simulink model "CryoDetHcd"  (R2016b)
settings: Solver=ode45  StartTime=0.0  StopTime=1e-3  RelTol=1e-3
PreLoadFcn:
  | setup_hcd
values from neighbouring files (symbols this model uses):
  A = sqrt(0.5*erfc(x))    [setup_hcd.m]
  Fadc = 307.2e6    (= 307200000)    [setupADCtoDACloopback.m]    (also in setupCryoFPGA_CMB.m; setup_hcd.m = 614000000)
undefined symbols (not defined in the file or in its folder): AXI4, B, C, D, etaRomData, freqRomData, freqRomData1, freqRomData2, freqRomData3, j, Lite
libraries: xbsIndex_r4 x897, CryoDetLibCMB x8, hdlsllib x8, dspsigops x2, simulink x1
(part 1 of 8)
settings Model: Creator=mdewart  LastModifiedBy=mdewart
settings DataIOCC: LimitDataPoints=on  SaveFormat=Array
settings OptimizationCC: BlockReduction=off  BooleanDataType=off  LifeSpan=inf
settings DebuggingCC: SaveWithParameterizedLinksMsg=none  UnderspecifiedInitializationDetection=Classic  MergeDetectMultiDrivingBlocksExec=none  SignalResolutionControl=TryResolveAllWithWarning  SFUnexpectedBacktrackingDiag=warning  SFNoUnconditionalDefaultTransitionDiag=warning  SFExecutionAtInitializationDiag=none
settings HardwareCC: ProdBitPerPointer=32  ProdBitPerSizeT=32  ProdBitPerPtrDiffT=32  ProdLargestAtomicFloat=None  ProdIntDivRoundTo=Undefined  ProdEndianess=Unspecified  ProdWordSize=32  ProdHWDeviceType=32-bit Generic  TargetUnknown=on
settings ModelReferenceCC: PropagateSignalLabelsOutOfModel=off
settings GRTTargetCC: TargetLangStandard=C89/C90 (ANSI)  GeneratePreprocessorConditionals=Disable all
settings ConfigComp: CovMetricSettings=dw  CovHtmlReporting=on  CovSaveCumulativeToWorkspaceVar=on  CovSaveSingleToWorkspaceVar=on  CovExternalEMLEnable=off  CovSFcnEnable=off

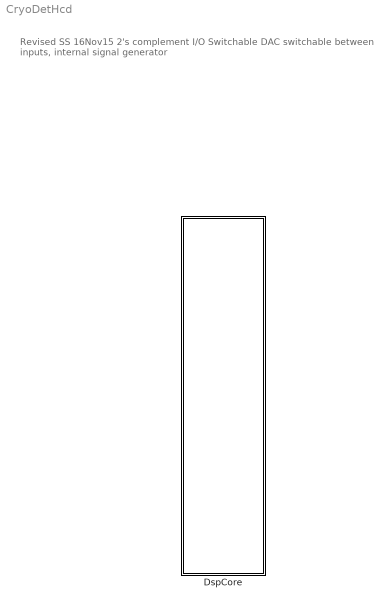
== system CryoDetHcd ==
  note: Revised SS 16Nov15
      | 	2's complement I/O
      | 	Switchable DAC switchable between inputs, internal signal generator
  DspCore : Subsystem

== system CryoDetHcd/DspCore ==
  " System Generator1" : xbsIndex_r4/ System Generator  Tag=genX  xilinxfamily=kintexu  part=xcku060  speed=-2-e  package=ffva1156  synthesis_tool=Vivado  clock_wrapper=Clock Enables  directory=./netlist  proj_type=Vivado  Synth_file=Vivado Synthesis Defaults  Impl_file=Vivado Implementation Defaults  testbench=off  simulink_period=2/Fadc  sysclk_period=2e9/Fadc  dcm_input_clock_period=10  incr_netlist=off  trim_vbits=Everywhere in SubSystem  dbl_ovrd=According to Block Masks  core_generation=According to Block Masks  run_coregen=off  deprecated_control=off  eval_field=0  block_type=sysgen
  DSP : Subsystem
  DSP_axi_lite : Subsystem
  Register{1..13} (13 alike) : xbsIndex_r4/Register  init=0  rst=off  en=off  dbl_ovrd=off  block_type=register
  tag scope: config0=global, config1=global, config2=global, config3=global, config4=global, config6=global, config7=global, config8=global, config=global
  wires:
  DSP_axi_lite/1(config0) -> Register2/1
  Register2/1 -> [config0]
  DSP_axi_lite/2(config1) -> Register1/1
  Register1/1 -> [config1]
  Register3/1 -> [config2]
  DSP_axi_lite/3(config2) -> Register3/1
  Register4/1 -> [config3]
  DSP_axi_lite/4(config3) -> Register4/1
  Register5/1 -> [config4]
  DSP_axi_lite/5(config4) -> Register5/1
  [IQ_status] -> Register6/1
  Register6/1 -> DSP_axi_lite/1(status1)
  [dspCounter] -> Register7/1
  Register7/1 -> DSP_axi_lite/2(status2)
  Register8/1 -> [config]
  DSP_axi_lite/6(config5) -> Register8/1
  [status] -> Register9/1
  Register9/1 -> DSP_axi_lite/3(status3)
  [analysis_IQ] -> Register10/1
  Register10/1 -> DSP_axi_lite/4(status4)
  Register11/1 -> [config6]
  DSP_axi_lite/7(config6) -> Register11/1
  Register12/1 -> [config7]
  DSP_axi_lite/8(config7) -> Register12/1
  DSP_axi_lite/9(config8) -> Register13/1
  Register13/1 -> [config8]

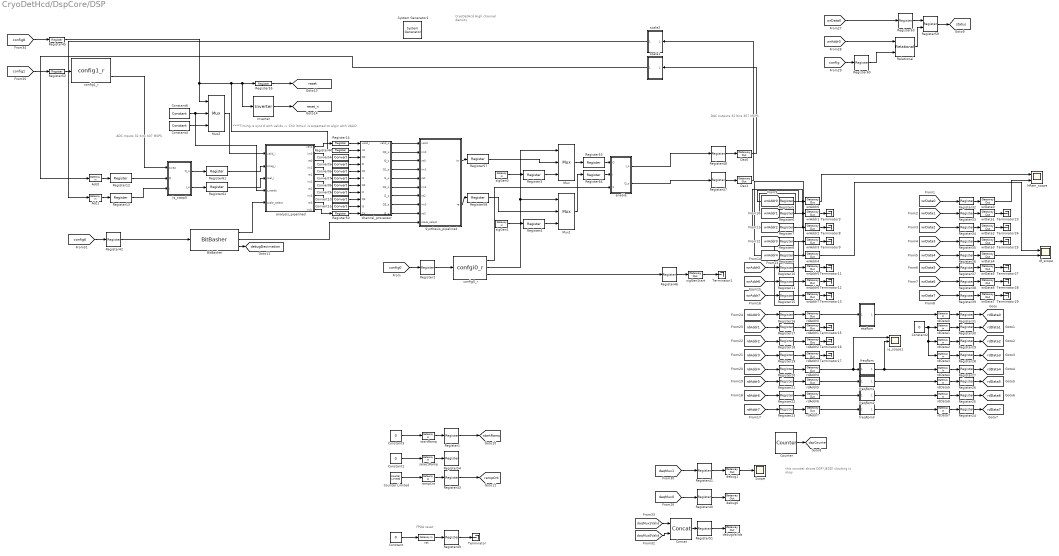
== system CryoDetHcd/DspCore/DSP ==
  note: this counter shows DSP (JESD) clocking
      | is okay
  note: ****Timing is sync'd with valids -> Ch0 (tmux) is expected to algin with VALID
  note: CryoDetHcd
      | High channel density
  note: DAC outputs
      | 32 bits
      | 307 MSPS
  note: ADC Inputs
      | 32 bits
      | 307 MSPS
  note: FPGA reset
  " System Generator1" : xbsIndex_r4/ System Generator  Tag=genX  xilinxfamily=kintexu  part=xcku060  speed=-2-e  package=ffva1156  synthesis_tool=Vivado  clock_wrapper=Clock Enables  directory=./netlist  proj_type=Vivado  Synth_file=Vivado Synthesis Defaults  Impl_file=Vivado Implementation Defaults  testbench=off  simulink_period=2/Fadc  sysclk_period=2e9/Fadc  dcm_input_clock_period=10  incr_netlist=off  trim_vbits=Everywhere in SubSystem  dbl_ovrd=According to Block Masks  core_generation=According to Block Masks  run_coregen=off  deprecated_control=off  eval_field=0  block_type=sysgen
  Adc0 : xbsIndex_r4/Gateway In  gui_display_data_type=Fixed-point  arith_type=Unsigned  n_bits=32  bin_pt=0  preci_type=Single  exp_width=8  frac_width=24  rows=1  columns=1  quantization=Truncate  overflow=Wrap  period=2/Fadc  UseAsADC=off  ADCChannel='1'  interface=None  automatic_assignment=on  address_offset=hex2dec('00')  intf_name=''  intf_description=''  default_value=0  timing_constraint=None  locs_specified=off  LOCs={}  io_standard={}  inherit_from_input=off  hdl_port=on  dbl_ovrd=off  block_type=gatewayin
  Adc1 : xbsIndex_r4/Gateway In  gui_display_data_type=Fixed-point  arith_type=Unsigned  n_bits=32  bin_pt=0  preci_type=Single  exp_width=8  frac_width=24  rows=1  columns=1  quantization=Truncate  overflow=Wrap  period=2/Fadc  UseAsADC=off  ADCChannel='1'  interface=None  automatic_assignment=on  address_offset=hex2dec('00')  intf_name=''  intf_description=''  default_value=0  timing_constraint=None  locs_specified=off  LOCs={}  io_standard={}  inherit_from_input=off  hdl_port=on  dbl_ovrd=off  block_type=gatewayin
  BitBasher : xbsIndex_r4/BitBasher  bitexpr=|  display_expr=off  sr_1=scale_analysis  arith_type1=Unsigned  bin_pt1=0  sr_2=scale_synthesis  arith_type2=Unsigned  bin_pt2=0  sr_3=debugDecimation  arith_type3=Unsigned  bin_pt3=0  sr_4=4  arith_type4=Unsigned  bin_pt4=0  dbl_ovrd=off  block_type=bitbasher
      | scale_analysis = {in[1:0]}
      | scale_synthesis = {in[3:2]}
      | debugDecimation = {in[6:4]}
  Concat : xbsIndex_r4/Concat  num_inputs=2  dbl_ovrd=off  block_type=concat
  Constant{,1..3} (4 alike) : Constant  Value=0
  Constant4 : xbsIndex_r4/Constant  const=0  gui_display_data_type=Boolean  arith_type=Boolean  n_bits=16  bin_pt=14  preci_type=Single  exp_width=8  frac_width=24  explicit_period=on  period=2/Fadc  equ=P=C  opselect=C  inp2=PCIN>>17  opr=+  inp1=P  carry=CIN  dbl_ovrd=off  block_type=constant
  Constant6 : xbsIndex_r4/Constant  const=1.0  gui_display_data_type=Boolean  arith_type=Boolean  n_bits=16  bin_pt=14  preci_type=Single  exp_width=8  frac_width=24  explicit_period=on  period=2/Fadc  equ=P=C  opselect=C  inp2=PCIN>>17  opr=+  inp1=P  carry=CIN  dbl_ovrd=off  block_type=constant
  Convert{4..11} (8 alike) : xbsIndex_r4/Convert  gui_display_data_type=Fixed-point  arith_type="Signed  (2's comp)"  n_bits=16  bin_pt=15  float_type=Single  exp_bits=8  fraction_bits=24  quantization=Truncate  overflow=Saturate  en=off  latency=1  pipeline=off  dbl_ovrd=off  block_type=convert
  Counter : xbsIndex_r4/Counter  cnt_type=Free Running  cnt_to=Inf  operation=Up  start_count=0  cnt_by_val=1  arith_type=Unsigned  n_bits=32  bin_pt=0  load_pin=off  rst=off  en=off  explicit_period=on  period=2/Fadc  use_behavioral_HDL=off  implementation=Fabric  dbl_ovrd=off  block_type=counter
  Counter Limited : simulink/Sources/Counter Limited  uplimit=2^32-1  tsamp=2/Fadc
  Dac0 : xbsIndex_r4/Gateway Out  inherit_from_input=on  hdl_port=on  rows=1  columns=1  UseAsDAC=off  DACChannel='1'  interface=None  automatic_assignment=on  address_offset=hex2dec('00')  intf_name=''  intf_description=''  timing_constraint=None  locs_specified=off  LOCs={}  io_standard={}  block_type=gatewayout
  Dac1 : xbsIndex_r4/Gateway Out  inherit_from_input=on  hdl_port=on  rows=1  columns=1  UseAsDAC=off  DACChannel='1'  interface=None  automatic_assignment=on  address_offset=hex2dec('00')  intf_name=''  intf_description=''  timing_constraint=None  locs_specified=off  LOCs={}  io_standard={}  block_type=gatewayout
  Inverter : xbsIndex_r4/Inverter  en=off  latency=1  dbl_ovrd=off  block_type=inv
  Mux : xbsIndex_r4/Mux  inputs=2  en=off  latency=1  precision=Full  arith_type=Unsigned  n_bits=16  bin_pt=14  quantization=Truncate  overflow=Wrap  dbl_ovrd=off  block_type=mux
  Mux1 : xbsIndex_r4/Mux  inputs=2  en=off  latency=1  precision=Full  arith_type=Unsigned  n_bits=16  bin_pt=14  quantization=Truncate  overflow=Wrap  dbl_ovrd=off  block_type=mux
  Mux2 : xbsIndex_r4/Mux  inputs=2  en=off  latency=1  precision=Full  arith_type=Unsigned  n_bits=16  bin_pt=14  quantization=Truncate  overflow=Wrap  dbl_ovrd=off  block_type=mux
  Register{1..55,57..58,60..64} (62 alike) : xbsIndex_r4/Register  init=0  rst=off  en=off  dbl_ovrd=off  block_type=register
  Register59 : xbsIndex_r4/Register  init=0  rst=off  en=on  dbl_ovrd=off  block_type=register
  Relational : xbsIndex_r4/Relational  mode=a=b  op_type=Bool  en=off  latency=1  dbl_ovrd=off  block_type=relational
  Scope : Scope
  Synthesis_pipelined : Subsystem  VariantControl=Variant
  Terminator{,1,3,8..9,11..13,15..17,23..25,27..29} (17 alike) : Terminator
  analysis_pipelined : Subsystem
  channel_processor : Subsystem  Variant=on  OverrideUsingVariant=Variant
  config0_r : CryoDetLibCMB/confgi0_r
  config1_r : CryoDetLibCMB/config1_r
  debug0 : xbsIndex_r4/Gateway Out  inherit_from_input=on  hdl_port=on  rows=1  columns=1  UseAsDAC=off  DACChannel='1'  interface=None  automatic_assignment=on  address_offset=hex2dec('00')  intf_name=''  intf_description=''  timing_constraint=None  locs_specified=off  LOCs={}  io_standard={}  block_type=gatewayout
  debug1 : xbsIndex_r4/Gateway Out  inherit_from_input=on  hdl_port=on  rows=1  columns=1  UseAsDAC=off  DACChannel='1'  interface=None  automatic_assignment=on  address_offset=hex2dec('00')  intf_name=''  intf_description=''  timing_constraint=None  locs_specified=off  LOCs={}  io_standard={}  block_type=gatewayout
  debugValids : xbsIndex_r4/Gateway Out  inherit_from_input=on  hdl_port=on  rows=1  columns=1  UseAsDAC=off  DACChannel='1'  interface=None  automatic_assignment=on  address_offset=hex2dec('00')  intf_name=''  intf_description=''  timing_constraint=None  locs_specified=off  LOCs={}  io_standard={}  block_type=gatewayout
  df_scope : Scope  NumInputPorts=2
  enable : Subsystem
  etaRom : Subsystem
  freqRom : Subsystem
  freqRom1 : Subsystem
  freqRom2 : Subsystem
  freqRom3 : Subsystem
  iq_scope1 : Scope  NumInputPorts=3
  iq_swap0 : Subsystem
  lrRam_scope : Scope  NumInputPorts=2
  rampCnt : xbsIndex_r4/Gateway In  gui_display_data_type=Fixed-point  arith_type=Unsigned  n_bits=32  bin_pt=0  preci_type=Single  exp_width=8  frac_width=24  rows=1  columns=1  quantization=Truncate  overflow=Wrap  period=2/Fadc  UseAsADC=off  ADCChannel='1'  interface=None  automatic_assignment=on  address_offset=hex2dec('00')  intf_name=''  intf_description=''  default_value=0  timing_constraint=None  locs_specified=off  LOCs={}  io_standard={}  inherit_from_input=off  hdl_port=on  dbl_ovrd=off  block_type=gatewayin
  rdAddr{0..7} (8 alike) : xbsIndex_r4/Gateway Out  inherit_from_input=on  hdl_port=on  rows=1  columns=1  UseAsDAC=off  DACChannel='1'  interface=None  automatic_assignment=on  address_offset=hex2dec('00')  intf_name=''  intf_description=''  timing_constraint=None  locs_specified=off  LOCs={}  io_standard={}  block_type=gatewayout
  rdData{0..7} (8 alike) : xbsIndex_r4/Gateway In  gui_display_data_type=Fixed-point  arith_type=Unsigned  n_bits=32  bin_pt=0  preci_type=Single  exp_width=8  frac_width=24  rows=1  columns=1  quantization=Truncate  overflow=Wrap  period=2/Fadc  UseAsADC=off  ADCChannel='1'  interface=None  automatic_assignment=on  address_offset=hex2dec('00')  intf_name=''  intf_description=''  default_value=0  timing_constraint=None  locs_specified=off  LOCs={}  io_standard={}  inherit_from_input=off  hdl_port=on  dbl_ovrd=off  block_type=gatewayin
  rst : xbsIndex_r4/Gateway In  gui_display_data_type=Boolean  arith_type=Boolean  n_bits=16  bin_pt=14  preci_type=Single  exp_width=8  frac_width=24  rows=1  columns=1  quantization="Round  (unbiased: +/- Inf)"  overflow=Saturate  period=2/Fadc  UseAsADC=off  ADCChannel='1'  interface=None  automatic_assignment=on  address_offset=hex2dec('00')  intf_name=''  intf_description=''  default_value=0  timing_constraint=None  locs_specified=off  LOCs={}  io_standard={}  inherit_from_input=off  hdl_port=on  dbl_ovrd=off  block_type=gatewayin
  scale1 : Subsystem
  scale2 : Subsystem
  selectRamp : xbsIndex_r4/Gateway In  gui_display_data_type=Boolean  arith_type=Boolean  n_bits=16  bin_pt=14  preci_type=Single  exp_width=8  frac_width=24  rows=1  columns=1  quantization=Truncate  overflow=Wrap  period=2/Fadc  UseAsADC=off  ADCChannel='1'  interface=None  automatic_assignment=on  address_offset=hex2dec('00')  intf_name=''  intf_description=''  default_value=0  timing_constraint=None  locs_specified=off  LOCs={}  io_standard={}  inherit_from_input=off  hdl_port=on  dbl_ovrd=off  block_type=gatewayin
  sigGen0 : xbsIndex_r4/Gateway In  gui_display_data_type=Fixed-point  arith_type=Unsigned  n_bits=32  bin_pt=0  preci_type=Single  exp_width=8  frac_width=24  rows=1  columns=1  quantization=Truncate  overflow=Wrap  period=2/Fadc  UseAsADC=off  ADCChannel='1'  interface=None  automatic_assignment=on  address_offset=hex2dec('00')  intf_name=''  intf_description=''  default_value=0  timing_constraint=None  locs_specified=off  LOCs={}  io_standard={}  inherit_from_input=off  hdl_port=on  dbl_ovrd=off  block_type=gatewayin
  sigGen1 : xbsIndex_r4/Gateway In  gui_display_data_type=Fixed-point  arith_type=Unsigned  n_bits=32  bin_pt=0  preci_type=Single  exp_width=8  frac_width=24  rows=1  columns=1  quantization=Truncate  overflow=Wrap  period=2/Fadc  UseAsADC=off  ADCChannel='1'  interface=None  automatic_assignment=on  address_offset=hex2dec('00')  intf_name=''  intf_description=''  default_value=0  timing_constraint=None  locs_specified=off  LOCs={}  io_standard={}  inherit_from_input=off  hdl_port=on  dbl_ovrd=off  block_type=gatewayin
  sigGenStart : xbsIndex_r4/Gateway Out  inherit_from_input=on  hdl_port=on  rows=1  columns=1  UseAsDAC=off  DACChannel='1'  interface=None  automatic_assignment=off  address_offset=hex2dec('004')  intf_name=''  intf_description=''  timing_constraint=None  locs_specified=off  LOCs={}  io_standard={}  block_type=gatewayout
  startRamp : xbsIndex_r4/Gateway In  gui_display_data_type=Boolean  arith_type=Boolean  n_bits=16  bin_pt=14  preci_type=Single  exp_width=8  frac_width=24  rows=1  columns=1  quantization=Truncate  overflow=Wrap  period=2/Fadc  UseAsADC=off  ADCChannel='1'  interface=None  automatic_assignment=on  address_offset=hex2dec('00')  intf_name=''  intf_description=''  default_value=0  timing_constraint=None  locs_specified=off  LOCs={}  io_standard={}  inherit_from_input=off  hdl_port=on  dbl_ovrd=off  block_type=gatewayin
  wrAddr{0..7} (8 alike) : xbsIndex_r4/Gateway Out  inherit_from_input=on  hdl_port=on  rows=1  columns=1  UseAsDAC=off  DACChannel='1'  interface=None  automatic_assignment=on  address_offset=hex2dec('00')  intf_name=''  intf_description=''  timing_constraint=None  locs_specified=off  LOCs={}  io_standard={}  block_type=gatewayout
  wrData{0..7} (8 alike) : xbsIndex_r4/Gateway Out  inherit_from_input=on  hdl_port=on  rows=1  columns=1  UseAsDAC=off  DACChannel='1'  interface=None  automatic_assignment=on  address_offset=hex2dec('00')  intf_name=''  intf_description=''  timing_constraint=None  locs_specified=off  LOCs={}  io_standard={}  block_type=gatewayout
  tag scope: debugDecimation=global, dspCounter=global, rampCnt=global, rdData0=global, rdData1=global, rdData2=global, rdData3=global, rdData4=global, rdData5=global, rdData6=global, rdData7=global, reset=global, reset_n=global, startRamp=global, status=global
  wires:
  startRamp/1 -> Register1/1
  Constant/1 -> rst/1
  rst/1 -> Register49/1
  sigGen0/1 -> Register3/1
  sigGen1/1 -> Register4/1
  sigGenStart/1 -> Terminator1/1
  [config0] -> Register2/1
  Register3/1 -> Mux/3
  Synthesis_pipelined/1(im) -> Register57/1
  Synthesis_pipelined/2(re) -> Register58/1
  analysis_pipelined/1(valid) -> Register14/1
  analysis_pipelined/2(im0) -> Convert4/1
  analysis_pipelined/3(re0) -> Convert5/1
  analysis_pipelined/4(im1) -> Convert6/1
  analysis_pipelined/5(re1) -> Convert7/1
  analysis_pipelined/6(im2) -> Convert8/1
  analysis_pipelined/7(re2) -> Convert9/1
  analysis_pipelined/8(im3) -> Convert10/1
  analysis_pipelined/9(re3) -> Convert11/1
  Adc0/1 -> Register12/1
  Adc1/1 -> Register13/1
  Register4/1 -> Mux1/3
  Register5/1 -> wrAddr0/1
  Register6/1 -> wrAddr1/1
  Register7/1 -> wrAddr2/1
  Register8/1 -> wrAddr3/1
  Register9/1 -> wrAddr4/1
  Register10/1 -> wrAddr5/1
  Register11/1 -> wrAddr6/1
  Register15/1 -> wrAddr7/1
  Register16/1 -> rdAddr0/1
  Register17/1 -> rdAddr1/1
  Register18/1 -> rdAddr2/1
  Register19/1 -> rdAddr3/1
  Register20/1 -> rdAddr4/1
  Register21/1 -> rdAddr5/1
  Register22/1 -> rdAddr6/1
  Register23/1 -> rdAddr7/1
  rdData7/1 -> Register24/1
  rdData3/1 -> Register28/1
  rdData4/1 -> Register27/1
  rdData5/1 -> Register26/1
  rdData6/1 -> Register25/1
  rdData2/1 -> Register29/1
  rdData1/1 -> Register30/1
  rdData0/1 -> Register31/1
  Register32/1 -> wrData0/1
  Register33/1 -> wrData1/1
  Register34/1 -> wrData2/1
  Register35/1 -> wrData3/1
  Register36/1 -> wrData4/1
  Register37/1 -> wrData5/1
  Register38/1 -> wrData6/1
  Register39/1 -> wrData7/1
  Register31/1 -> [rdData0]
  Register30/1 -> [rdData1]
  Register28/1 -> [rdData3]
  Register27/1 -> [rdData4]
  Register25/1 -> [rdData6]
  Register24/1 -> [rdData7]
  Register29/1 -> [rdData2]
  [wrData0] -> Register32/1
  [wrData7] -> Register39/1
  [wrData6] -> Register38/1
  [wrData5] -> Register37/1
  [wrData4] -> Register36/1
  [wrData3] -> Register35/1
  [wrData2] -> Register34/1
  [wrData1] -> Register33/1
  [wrAddr7] -> Register15/1
  [wrAddr6] -> Register11/1
  [wrAddr5] -> Register10/1
  [wrAddr4] -> Register9/1
  [wrAddr3] -> Register8/1
  [wrAddr2] -> Register7/1
  [wrAddr1] -> Register6/1
  [wrAddr0] -> Register5/1
  [rdAddr7] -> Register23/1
  [rdAddr6] -> Register22/1
  [rdAddr5] -> Register21/1
  [rdAddr4] -> Register20/1
  [rdAddr3] -> Register19/1
  [rdAddr2] -> Register18/1
  [rdAddr1] -> Register17/1
  [rdAddr0] -> Register16/1
  wrAddr1/1 -> Terminator3/1
  wrAddr2/1 -> Terminator8/1
  wrAddr3/1 -> Terminator9/1
  wrAddr4/1 -> df_scope/1
  wrAddr5/1 -> Terminator11/1
  wrAddr6/1 -> Terminator12/1
  wrAddr7/1 -> Terminator13/1
  rdAddr1/1 -> Terminator15/1
  rdAddr2/1 -> Terminator16/1
  rdAddr3/1 -> Terminator17/1
  wrData1/1 -> Terminator23/1
  wrData2/1 -> Terminator24/1
  wrData3/1 -> Terminator25/1
  wrData5/1 -> Terminator27/1
  wrData6/1 -> Terminator28/1
  wrData7/1 -> Terminator29/1
  Constant2/1 -> rdData1/1, rdData2/1, rdData3/1
  Register26/1 -> [rdData5]
  Register40/1 -> debug0/1
  Register41/1 -> debug1/1
  Register47/1 -> Dac1/1
  Register48/1 -> Dac0/1
  Register49/1 -> Terminator/1
  Constant3/1 -> startRamp/1
  analysis_pipelined/10(indx) -> Register50/1
  Register51/1 -> debugValids/1
  [config1] -> Register52/1
  Register46/1 -> sigGenStart/1
  Mux/1 -> Register53/1
  config0_r/2 -> Mux1/1, Mux/1
  Register2/1 -> config0_r/1
  config0_r/3 -> Register46/1
  Register52/1 -> config1_r/1
  config1_r/2 -> iq_swap0/1(swap)
  Register12/1 -> iq_swap0/2(Q)
  Register13/1 -> iq_swap0/3(I)
  iq_swap0/1(Q_o) -> Register61/1
  iq_swap0/2(I_o) -> Register62/1
  Counter/1 -> [dspCounter]
  Convert7/1 -> channel_processor/6(I1)
  Convert5/1 -> channel_processor/4(I0)
  Convert10/1 -> channel_processor/9(Q3)
  Convert11/1 -> channel_processor/10(I3)
  Register50/1 -> channel_processor/11(Ch)
  Register14/1 -> channel_processor/1(valid_i)
  Convert9/1 -> channel_processor/8(I2)
  Convert6/1 -> channel_processor/5(Q1)
  Convert4/1 -> channel_processor/3(Q0)
  Convert8/1 -> channel_processor/7(Q2)
  channel_processor/5(I1_o) -> Synthesis_pipelined/5(re1)
  channel_processor/4(Q1_o) -> Synthesis_pipelined/4(im1)
  channel_processor/6(Q2_o) -> Synthesis_pipelined/6(im2)
  channel_processor/7(I2_o) -> Synthesis_pipelined/7(re2)
  channel_processor/8(Q3_o) -> Synthesis_pipelined/8(im3)
  channel_processor/1(valid_o) -> Synthesis_pipelined/1(valid)
  channel_processor/9(I3_o) -> Synthesis_pipelined/9(re3)
  channel_processor/2(Q0_o) -> Synthesis_pipelined/2(im0)
  channel_processor/3(I0_o) -> Synthesis_pipelined/3(re0)
  Register53/1 -> enable/1(Q)
  config0_r/1 -> enable/3(enable)
  Register57/1 -> Mux/2
  Register58/1 -> Mux1/2
  rdAddr4/1 -> iq_scope1/1, freqRom/1(In1)
  freqRom/1(Out1) -> iq_scope1/2, rdData4/1
  wrAddr0/1 -> lrRam_scope/1
  wrData0/1 -> lrRam_scope/2
  wrData4/1 -> df_scope/2
  [wrAddr0] -> Relational/1
  [wrData0] -> Register63/1
  Register59/1 -> [status]
  Register60/1 -> Relational/2
  [config] -> Register60/1
  Register61/1 -> analysis_pipelined/2(imag_i)
  Register62/1 -> analysis_pipelined/3(real_i)
  Relational/1 -> Register59/2
  Register63/1 -> Register59/1
  Dac0/1 -> scale1/1(In1)
  Dac1/1 -> scale2/1(In1)
  scale1/1(Out1) -> Adc0/1
  scale2/1(Out1) -> Adc1/1
  enable/1(I_o) -> Register48/1
  enable/2(Q_o) -> Register47/1
  etaRom/1(Out1) -> rdData0/1
  rdAddr0/1 -> etaRom/1(In1)
  Mux1/1 -> Register64/1
  Register64/1 -> enable/2(I)
  selectRamp/1 -> Register54/1
  Constant1/1 -> selectRamp/1
  Register1/1 -> [startRamp]
  [daqMux0] -> Register40/1
  [daqMux1] -> Register41/1
  [config6] -> Register42/1
  Register42/1 -> BitBasher/1
  BitBasher/2 -> Synthesis_pipelined/10(scale_select)
  BitBasher/1 -> analysis_pipelined/5(scale_select)
  [daqMux1Valid] -> Concat/1
  Concat/1 -> Register51/1
  [daqMux0Valid] -> Concat/2
  BitBasher/3 -> [debugDecimation]
  rampCnt/1 -> Register43/1
  Register43/1 -> [rampCnt]
  rdAddr5/1 -> freqRom1/1(In1)
  freqRom1/1(Out1) -> rdData5/1
  rdAddr6/1 -> freqRom2/1(In1)
  freqRom2/1(Out1) -> rdData6/1
  rdAddr7/1 -> freqRom3/1(In1)
  freqRom3/1(Out1) -> rdData7/1
  debug1/1 -> Scope/1
  Counter Limited/1 -> rampCnt/1
  Register45/1 -> Mux2/1, Register55/1, Inverter/1, Register44/1
  Constant6/1 -> Mux2/2, analysis_pipelined/4(t_ready)
  Mux2/1 -> analysis_pipelined/1(valid_i)
  Constant4/1 -> Mux2/3
  Register44/1 -> channel_processor/2(rst)
  [config8] -> Register45/1
  Inverter/1 -> [reset_n]
  Register55/1 -> [reset]

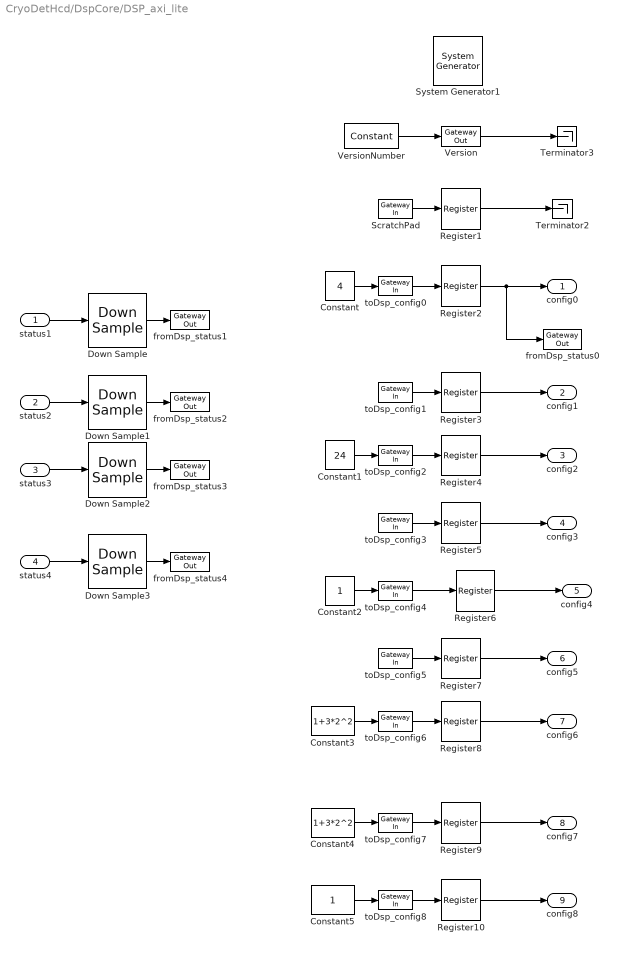
== system CryoDetHcd/DspCore/DSP_axi_lite ==
  status1 : Inport
  status2 : Inport  Port=2
  status3 : Inport  Port=3
  status4 : Inport  Port=4
  " System Generator1" : xbsIndex_r4/ System Generator  Tag=genX  xilinxfamily=kintexu  part=xcku060  speed=-2-e  package=ffva1156  synthesis_tool=Vivado  clock_wrapper=Clock Enables  directory=./netlist  proj_type=Vivado  Synth_file=Vivado Synthesis Defaults  Impl_file=Vivado Implementation Defaults  testbench=off  simulink_period=1/156.25e6  sysclk_period=1e9/(156.25e6)  dcm_input_clock_period=10  incr_netlist=off  trim_vbits=Everywhere in SubSystem  dbl_ovrd=According to Block Masks  core_generation=According to Block Masks  run_coregen=off  deprecated_control=off  eval_field=0  block_type=sysgen
  Constant : Constant  Value=4
  Constant1 : Constant  Value=24
  Constant2 : Constant
  Constant3 : Constant  Value=1+3*2^2
  Constant4 : Constant  Value=1+3*2^2
  Constant5 : Constant
  Down Sample{,1..3} (4 alike) : xbsIndex_r4/Down Sample  sample_ratio=16  sample_phase="Last Value of Frame  (most efficient)"  en=off  rst=off  latency=1  dbl_ovrd=off  block_type=dsamp
  Register{1..10} (10 alike) : xbsIndex_r4/Register  init=0  rst=off  en=off  dbl_ovrd=off  block_type=register
  ScratchPad : xbsIndex_r4/Gateway In  gui_display_data_type=Fixed-point  arith_type=Unsigned  n_bits=32  bin_pt=0  preci_type=Single  exp_width=8  frac_width=24  rows=1  columns=1  quantization="Round  (unbiased: +/- Inf)"  overflow=Saturate  period=16/156.25e6  UseAsADC=off  ADCChannel='1'  interface=AXI4-Lite  automatic_assignment=off  address_offset=hex2dec('FFC')  intf_name=''  intf_description=''  default_value=0  timing_constraint=None  locs_specified=off  LOCs={}  io_standard={}  inherit_from_input=off  hdl_port=on  dbl_ovrd=off  block_type=gatewayin
  Terminator2 : Terminator
  Terminator3 : Terminator
  Version : xbsIndex_r4/Gateway Out  inherit_from_input=on  hdl_port=on  rows=1  columns=1  UseAsDAC=off  DACChannel='1'  interface=AXI4-Lite  automatic_assignment=off  address_offset=hex2dec('000')  intf_name=''  intf_description=''  timing_constraint=None  locs_specified=off  LOCs={}  io_standard={}  block_type=gatewayout
  VersionNumber : xbsIndex_r4/Constant  const=hex2dec('00000001')  gui_display_data_type=Fixed-point  arith_type=Unsigned  n_bits=32  bin_pt=0  preci_type=Single  exp_width=8  frac_width=24  explicit_period=on  period=16/156.25e6  equ=P=C  opselect=C  inp2=PCIN>>17  opr=+  inp1=P  carry=CIN  dbl_ovrd=off  block_type=constant
  fromDsp_status0 : xbsIndex_r4/Gateway Out  inherit_from_input=on  hdl_port=on  rows=1  columns=1  UseAsDAC=off  DACChannel='1'  interface=AXI4-Lite  automatic_assignment=off  address_offset=hex2dec('004')  intf_name=''  intf_description=''  timing_constraint=None  locs_specified=off  LOCs={}  io_standard={}  block_type=gatewayout
  fromDsp_status1 : xbsIndex_r4/Gateway Out  inherit_from_input=on  hdl_port=on  rows=1  columns=1  UseAsDAC=off  DACChannel='1'  interface=AXI4-Lite  automatic_assignment=off  address_offset=hex2dec('008')  intf_name=''  intf_description=''  timing_constraint=None  locs_specified=off  LOCs={}  io_standard={}  block_type=gatewayout
  fromDsp_status2 : xbsIndex_r4/Gateway Out  inherit_from_input=on  hdl_port=on  rows=1  columns=1  UseAsDAC=off  DACChannel='1'  interface=AXI4-Lite  automatic_assignment=off  address_offset=hex2dec('00C')  intf_name=''  intf_description=''  timing_constraint=None  locs_specified=off  LOCs={}  io_standard={}  block_type=gatewayout
  fromDsp_status3 : xbsIndex_r4/Gateway Out  inherit_from_input=on  hdl_port=on  rows=1  columns=1  UseAsDAC=off  DACChannel='1'  interface=AXI4-Lite  automatic_assignment=off  address_offset=hex2dec('010')  intf_name=''  intf_description=''  timing_constraint=None  locs_specified=off  LOCs={}  io_standard={}  block_type=gatewayout
  fromDsp_status4 : xbsIndex_r4/Gateway Out  inherit_from_input=on  hdl_port=on  rows=1  columns=1  UseAsDAC=off  DACChannel='1'  interface=AXI4-Lite  automatic_assignment=off  address_offset=hex2dec('014')  intf_name=''  intf_description=''  timing_constraint=None  locs_specified=off  LOCs={}  io_standard={}  block_type=gatewayout
  toDsp_config0 : xbsIndex_r4/Gateway In  gui_display_data_type=Fixed-point  arith_type=Unsigned  n_bits=32  bin_pt=0  preci_type=Single  exp_width=8  frac_width=24  rows=1  columns=1  quantization="Round  (unbiased: +/- Inf)"  overflow=Saturate  period=16/156.25e6  UseAsADC=off  ADCChannel='1'  interface=AXI4-Lite  automatic_assignment=off  address_offset=hex2dec('080')  intf_name=''  intf_description=''  default_value=0  timing_constraint=None  locs_specified=off  LOCs={}  io_standard={}  inherit_from_input=off  hdl_port=on  dbl_ovrd=off  block_type=gatewayin
  toDsp_config1 : xbsIndex_r4/Gateway In  gui_display_data_type=Fixed-point  arith_type=Unsigned  n_bits=32  bin_pt=0  preci_type=Single  exp_width=8  frac_width=24  rows=1  columns=1  quantization="Round  (unbiased: +/- Inf)"  overflow=Saturate  period=16/156.25e6  UseAsADC=off  ADCChannel='1'  interface=AXI4-Lite  automatic_assignment=off  address_offset=hex2dec('084')  intf_name=''  intf_description=''  default_value=0  timing_constraint=None  locs_specified=off  LOCs={}  io_standard={}  inherit_from_input=off  hdl_port=on  dbl_ovrd=off  block_type=gatewayin
  toDsp_config2 : xbsIndex_r4/Gateway In  gui_display_data_type=Fixed-point  arith_type=Unsigned  n_bits=32  bin_pt=0  preci_type=Single  exp_width=8  frac_width=24  rows=1  columns=1  quantization="Round  (unbiased: +/- Inf)"  overflow=Saturate  period=16/156.25e6  UseAsADC=off  ADCChannel='1'  interface=AXI4-Lite  automatic_assignment=off  address_offset=hex2dec('088')  intf_name=''  intf_description=''  default_value=0  timing_constraint=None  locs_specified=off  LOCs={}  io_standard={}  inherit_from_input=off  hdl_port=on  dbl_ovrd=off  block_type=gatewayin
  toDsp_config3 : xbsIndex_r4/Gateway In  gui_display_data_type=Fixed-point  arith_type=Unsigned  n_bits=32  bin_pt=0  preci_type=Single  exp_width=8  frac_width=24  rows=1  columns=1  quantization="Round  (unbiased: +/- Inf)"  overflow=Saturate  period=16/156.25e6  UseAsADC=off  ADCChannel='1'  interface=AXI4-Lite  automatic_assignment=off  address_offset=hex2dec('08C')  intf_name=''  intf_description=''  default_value=0  timing_constraint=None  locs_specified=off  LOCs={}  io_standard={}  inherit_from_input=off  hdl_port=on  dbl_ovrd=off  block_type=gatewayin
  toDsp_config4 : xbsIndex_r4/Gateway In  gui_display_data_type=Fixed-point  arith_type=Unsigned  n_bits=16  bin_pt=15  preci_type=Single  exp_width=8  frac_width=24  rows=1  columns=1  quantization="Round  (unbiased: +/- Inf)"  overflow=Saturate  period=16/156.25e6  UseAsADC=off  ADCChannel='1'  interface=AXI4-Lite  automatic_assignment=off  address_offset=hex2dec('090')  intf_name=''  intf_description=''  default_value=0  timing_constraint=None  locs_specified=off  LOCs={}  io_standard={}  inherit_from_input=off  hdl_port=on  dbl_ovrd=off  block_type=gatewayin
  toDsp_config5 : xbsIndex_r4/Gateway In  gui_display_data_type=Fixed-point  arith_type=Unsigned  n_bits=7  bin_pt=0  preci_type=Single  exp_width=8  frac_width=24  rows=1  columns=1  quantization="Round  (unbiased: +/- Inf)"  overflow=Saturate  period=16/156.25e6  UseAsADC=off  ADCChannel='1'  interface=AXI4-Lite  automatic_assignment=off  address_offset=hex2dec('094')  intf_name=''  intf_description=''  default_value=0  timing_constraint=None  locs_specified=off  LOCs={}  io_standard={}  inherit_from_input=off  hdl_port=on  dbl_ovrd=off  block_type=gatewayin
  toDsp_config6 : xbsIndex_r4/Gateway In  gui_display_data_type=Fixed-point  arith_type=Unsigned  n_bits=32  bin_pt=0  preci_type=Single  exp_width=8  frac_width=24  rows=1  columns=1  quantization="Round  (unbiased: +/- Inf)"  overflow=Saturate  period=16/156.25e6  UseAsADC=off  ADCChannel='1'  interface=AXI4-Lite  automatic_assignment=off  address_offset=hex2dec('098')  intf_name=''  intf_description=''  default_value=0  timing_constraint=None  locs_specified=off  LOCs={}  io_standard={}  inherit_from_input=off  hdl_port=on  dbl_ovrd=off  block_type=gatewayin
  toDsp_config7 : xbsIndex_r4/Gateway In  gui_display_data_type=Fixed-point  arith_type=Unsigned  n_bits=32  bin_pt=0  preci_type=Single  exp_width=8  frac_width=24  rows=1  columns=1  quantization="Round  (unbiased: +/- Inf)"  overflow=Saturate  period=16/156.25e6  UseAsADC=off  ADCChannel='1'  interface=AXI4-Lite  automatic_assignment=off  address_offset=hex2dec('09C')  intf_name=''  intf_description=''  default_value=0  timing_constraint=None  locs_specified=off  LOCs={}  io_standard={}  inherit_from_input=off  hdl_port=on  dbl_ovrd=off  block_type=gatewayin
  toDsp_config8 : xbsIndex_r4/Gateway In  gui_display_data_type=Boolean  arith_type=Boolean  n_bits=1  bin_pt=0  preci_type=Single  exp_width=8  frac_width=24  rows=1  columns=1  quantization="Round  (unbiased: +/- Inf)"  overflow=Saturate  period=16/156.25e6  UseAsADC=off  ADCChannel='1'  interface=AXI4-Lite  automatic_assignment=off  address_offset=hex2dec('100')  intf_name=''  intf_description=''  default_value=1  timing_constraint=None  locs_specified=off  LOCs={}  io_standard={}  inherit_from_input=off  hdl_port=on  dbl_ovrd=off  block_type=gatewayin
  config0 : Outport
  config1 : Outport  Port=2
  config2 : Outport  Port=3
  config3 : Outport  Port=4
  config4 : Outport  Port=5
  config5 : Outport  Port=6
  config6 : Outport  Port=7
  config7 : Outport  Port=8
  config8 : Outport  Port=9
  wires:
  toDsp_config0/1 -> Register2/1
  Register2/1 -> config0/1, fromDsp_status0/1
  ScratchPad/1 -> Register1/1
  Version/1 -> Terminator3/1
  VersionNumber/1 -> Version/1
  Register1/1 -> Terminator2/1
  toDsp_config1/1 -> Register3/1
  Register3/1 -> config1/1
  toDsp_config2/1 -> Register4/1
  Register4/1 -> config2/1
  toDsp_config3/1 -> Register5/1
  Register5/1 -> config3/1
  toDsp_config4/1 -> Register6/1
  Register6/1 -> config4/1
  status1/1 -> Down Sample/1
  Down Sample/1 -> fromDsp_status1/1
  status2/1 -> Down Sample1/1
  Down Sample1/1 -> fromDsp_status2/1
  status3/1 -> Down Sample2/1
  Down Sample2/1 -> fromDsp_status3/1
  toDsp_config5/1 -> Register7/1
  Register7/1 -> config5/1
  Constant/1 -> toDsp_config0/1
  Constant1/1 -> toDsp_config2/1
  status4/1 -> Down Sample3/1
  Down Sample3/1 -> fromDsp_status4/1
  Constant2/1 -> toDsp_config4/1
  toDsp_config6/1 -> Register8/1
  Register8/1 -> config6/1
  Constant3/1 -> toDsp_config6/1
  toDsp_config7/1 -> Register9/1
  Register9/1 -> config7/1
  Constant4/1 -> toDsp_config7/1
  toDsp_config8/1 -> Register10/1
  Register10/1 -> config8/1
  Constant5/1 -> toDsp_config8/1

== system CryoDetHcd/DspCore/DSP/Synthesis_pipelined ==
  note: TODO check scale values at bitbashers in synth
  valid : Inport
  im0 : Inport  Port=2
  re0 : Inport  Port=3
  im1 : Inport  Port=4
  re1 : Inport  Port=5
  im2 : Inport  Port=6
  re2 : Inport  Port=7
  im3 : Inport  Port=8
  re3 : Inport  Port=9
  scale_select : Inport  Port=10
  Synthesis : Subsystem
  im : Outport
  re : Outport  Port=2
  wires:
  valid/1 -> Synthesis/1(valid)
  im0/1 -> Synthesis/2(im0)
  im1/1 -> Synthesis/4(im1)
  re2/1 -> Synthesis/7(re2)
  re3/1 -> Synthesis/9(re3)
  re0/1 -> Synthesis/3(re0)
  re1/1 -> Synthesis/5(re1)
  im2/1 -> Synthesis/6(im2)
  im3/1 -> Synthesis/8(im3)
  Synthesis/2(re) -> re/1
  Synthesis/1(im) -> im/1
  scale_select/1 -> Synthesis/10(scale_select)

== system CryoDetHcd/DspCore/DSP/analysis_pipelined ==
  valid_i : Inport
  imag_i : Inport  Port=2
  real_i : Inport  Port=3
  t_ready : Inport  Port=4
  scale_select : Inport  Port=5
  Analysis0 : Subsystem
  Analysis1 : Subsystem
  Demux : Demux  Outputs=8
  Enabled Subsystem : Subsystem  TreatAsAtomicUnit=on
  Gateway Out : xbsIndex_r4/Gateway Out  inherit_from_input=off  hdl_port=off  rows=1  columns=1  UseAsDAC=off  DACChannel='1'  interface=None  automatic_assignment=on  address_offset=hex2dec('00')  intf_name=''  intf_description=''  timing_constraint=None  locs_specified=off  LOCs={}  io_standard={}  block_type=gatewayout
  Gateway Out1 : xbsIndex_r4/Gateway Out  inherit_from_input=off  hdl_port=off  rows=1  columns=1  UseAsDAC=off  DACChannel='1'  interface=None  automatic_assignment=on  address_offset=hex2dec('00')  intf_name=''  intf_description=''  timing_constraint=None  locs_specified=off  LOCs={}  io_standard={}  block_type=gatewayout
  Pre-Analysis0 : Subsystem
  Pre-Analysis1 : Subsystem
  Real-Imag to Complex2 : RealImagToComplex
  Scope : Scope  NumInputPorts=8
  valid : Outport
  im0 : Outport  Port=2
  re0 : Outport  Port=3
  im1 : Outport  Port=4
  re1 : Outport  Port=5
  im2 : Outport  Port=6
  re2 : Outport  Port=7
  im3 : Outport  Port=8
  re3 : Outport  Port=9
  indx : Outport  Port=10
  wires:
  Analysis0/5(valid1) -> Enabled Subsystem/Enable
  Analysis0/6(re1) -> im1/1
  Analysis0/7(im1) -> re1/1
  Demux/1 -> Scope/1
  Demux/2 -> Scope/2
  Demux/3 -> Scope/3
  Demux/4 -> Scope/4
  Demux/5 -> Scope/5
  Demux/6 -> Scope/6
  Demux/7 -> Scope/7
  Demux/8 -> Scope/8
  Enabled Subsystem/1(Out1) -> Demux/1
  Gateway Out1/1 -> Real-Imag to Complex2/1
  Gateway Out/1 -> Real-Imag to Complex2/2
  Real-Imag to Complex2/1 -> Enabled Subsystem/1(In1)
  Analysis1/7(im1) -> re3/1, Gateway Out/1
  Analysis1/6(re1) -> im3/1, Gateway Out1/1
  Analysis1/3(im0) -> re2/1
  Analysis1/2(re0) -> im2/1
  Analysis0/1(valid0) -> valid/1
  Analysis0/2(re0) -> im0/1
  Analysis0/3(im0) -> re0/1
  Pre-Analysis0/3(reo) -> Analysis0/3(In3)
  Pre-Analysis0/2(im0) -> Analysis0/2(In2)
  Pre-Analysis0/1(valid0) -> Analysis0/1(In1)
  t_ready/1 -> Analysis1/4(t_ready), Analysis0/4(t_ready)
  Pre-Analysis1/1(valid0) -> Analysis1/1(In1)
  valid_i/1 -> Pre-Analysis0/1(valid), Pre-Analysis1/1(valid)
  real_i/1 -> Pre-Analysis1/3(re), Pre-Analysis0/3(re)
  imag_i/1 -> Pre-Analysis1/2(im), Pre-Analysis0/2(im)
  Analysis0/4(indx0) -> indx/1
  Pre-Analysis1/2(im0) -> Analysis1/2(In2)
  Pre-Analysis1/3(reo) -> Analysis1/3(In3)
  scale_select/1 -> Analysis1/5(sel_scale), Analysis0/5(sel_scale)

== system CryoDetHcd/DspCore/DSP/channel_processor ==
  note: 1) Add Subsystem or Model blocks as valid variant choices.
      | 2) You cannot connect blocks at this level. At simulation, connectivity is automatically
      | determined, based on the active variant and port name matching.
  valid_i : Inport
  rst : Inport  Port=2
  Q0 : Inport  Port=3
  I0 : Inport  Port=4
  Q1 : Inport  Port=5
  I1 : Inport  Port=6
  Q2 : Inport  Port=7
  I2 : Inport  Port=8
  Q3 : Inport  Port=9
  I3 : Inport  Port=10
  Ch : Inport  Port=11
  channel_processor_x1 : Subsystem  VariantControl=Variant1
  channel_processor_x4 : Subsystem  VariantControl=Variant
  valid_o : Outport
  Q0_o : Outport  Port=2
  I0_o : Outport  Port=3
  Q1_o : Outport  Port=4
  I1_o : Outport  Port=5
  Q2_o : Outport  Port=6
  I2_o : Outport  Port=7
  Q3_o : Outport  Port=8
  I3_o : Outport  Port=9

== system CryoDetHcd/DspCore/DSP/enable ==
  Q : Inport
  I : Inport  Port=2
  enable : Inport  Port=3
  Constant7 : xbsIndex_r4/Constant  const=0  gui_display_data_type=Fixed-point  arith_type=Unsigned  n_bits=32  bin_pt=0  preci_type=Single  exp_width=8  frac_width=24  explicit_period=off  period=1  equ=P=C  opselect=C  inp2=PCIN>>17  opr=+  inp1=P  carry=CIN  dbl_ovrd=off  block_type=constant
  Mux2 : xbsIndex_r4/Mux  inputs=2  en=off  latency=1  precision=Full  arith_type=Unsigned  n_bits=16  bin_pt=14  quantization=Truncate  overflow=Wrap  dbl_ovrd=off  block_type=mux
  Mux3 : xbsIndex_r4/Mux  inputs=2  en=off  latency=1  precision=Full  arith_type=Unsigned  n_bits=16  bin_pt=14  quantization=Truncate  overflow=Wrap  dbl_ovrd=off  block_type=mux
  I_o : Outport
  Q_o : Outport  Port=2
  wires:
  Mux3/1 -> Q_o/1
  Mux2/1 -> I_o/1
  I/1 -> Mux3/3
  Q/1 -> Mux2/3
  enable/1 -> Mux3/1, Mux2/1
  Constant7/1 -> Mux3/2, Mux2/2

== system CryoDetHcd/DspCore/DSP/etaRom ==
  In1 : Inport
  1-D Lookup Table : Lookup_n-D  NumberOfTableDimensions=1  BreakpointsSpecification=Even spacing  BreakpointsForDimension1=[-5:5]  Table=etaRomData  InterpMethod=Nearest  InternalRulePriority=Speed  OutDataTypeStr=uint32  RndMeth=Simplest  InputSameDT=on
  Add : Sum
  Constant16 : Constant
  Delay9 : Delay  InitialCondition=0
  Out1 : Outport
  wires:
  Delay9/1 -> Add/1
  Constant16/1 -> Add/2
  Add/1 -> 1-D Lookup Table/1
  1-D Lookup Table/1 -> Out1/1
  In1/1 -> Delay9/1

== system CryoDetHcd/DspCore/DSP/freqRom ==
  In1 : Inport
  1-D Lookup Table : Lookup_n-D  NumberOfTableDimensions=1  BreakpointsSpecification=Even spacing  BreakpointsForDimension1=[-5:5]  Table=freqRomData  InterpMethod=Nearest  InternalRulePriority=Speed  OutDataTypeStr=uint32  RndMeth=Simplest  InputSameDT=on
  Add : Sum
  Constant16 : Constant
  Delay9 : Delay  InitialCondition=0
  Out1 : Outport
  wires:
  In1/1 -> Delay9/1
  1-D Lookup Table/1 -> Out1/1
  Add/1 -> 1-D Lookup Table/1
  Constant16/1 -> Add/2
  Delay9/1 -> Add/1

== system CryoDetHcd/DspCore/DSP/freqRom1 ==
  In1 : Inport
  1-D Lookup Table : Lookup_n-D  NumberOfTableDimensions=1  BreakpointsSpecification=Even spacing  BreakpointsForDimension1=[-5:5]  Table=freqRomData1  InterpMethod=Nearest  InternalRulePriority=Speed  OutDataTypeStr=uint32  RndMeth=Simplest  InputSameDT=on
  Add : Sum
  Constant16 : Constant
  Delay9 : Delay  InitialCondition=0
  Out1 : Outport
  wires:
  Delay9/1 -> Add/1
  Constant16/1 -> Add/2
  Add/1 -> 1-D Lookup Table/1
  1-D Lookup Table/1 -> Out1/1
  In1/1 -> Delay9/1

== system CryoDetHcd/DspCore/DSP/freqRom2 ==
  In1 : Inport
  1-D Lookup Table : Lookup_n-D  NumberOfTableDimensions=1  BreakpointsSpecification=Even spacing  BreakpointsForDimension1=[-5:5]  Table=freqRomData2  InterpMethod=Nearest  InternalRulePriority=Speed  OutDataTypeStr=uint32  RndMeth=Simplest  InputSameDT=on
  Add : Sum
  Constant16 : Constant
  Delay9 : Delay  InitialCondition=0
  Out1 : Outport
  wires:
  In1/1 -> Delay9/1
  1-D Lookup Table/1 -> Out1/1
  Add/1 -> 1-D Lookup Table/1
  Constant16/1 -> Add/2
  Delay9/1 -> Add/1

== system CryoDetHcd/DspCore/DSP/freqRom3 ==
  In1 : Inport
  1-D Lookup Table : Lookup_n-D  NumberOfTableDimensions=1  BreakpointsSpecification=Even spacing  BreakpointsForDimension1=[-5:5]  Table=freqRomData3  InterpMethod=Nearest  InternalRulePriority=Speed  OutDataTypeStr=uint32  RndMeth=Simplest  InputSameDT=on
  Add : Sum
  Constant16 : Constant
  Delay9 : Delay  InitialCondition=0
  Out1 : Outport
  wires:
  Delay9/1 -> Add/1
  Constant16/1 -> Add/2
  Add/1 -> 1-D Lookup Table/1
  1-D Lookup Table/1 -> Out1/1
  In1/1 -> Delay9/1

== system CryoDetHcd/DspCore/DSP/iq_swap0 ==
  swap : Inport
  Q : Inport  Port=2
  I : Inport  Port=3
  Mux4 : xbsIndex_r4/Mux  inputs=2  en=off  latency=1  precision=Full  arith_type=Unsigned  n_bits=16  bin_pt=14  quantization=Truncate  overflow=Wrap  dbl_ovrd=off  block_type=mux
  Mux5 : xbsIndex_r4/Mux  inputs=2  en=off  latency=1  precision=Full  arith_type=Unsigned  n_bits=16  bin_pt=14  quantization=Truncate  overflow=Wrap  dbl_ovrd=off  block_type=mux
  Q_o : Outport
  I_o : Outport  Port=2
  wires:
  Mux4/1 -> Q_o/1
  Mux5/1 -> I_o/1
  Q/1 -> Mux4/2, Mux5/3
  swap/1 -> Mux5/1, Mux4/1
  I/1 -> Mux5/2, Mux4/3

== system CryoDetHcd/DspCore/DSP/scale1 ==
  In1 : Inport
  Bit Concat : hdlsllib/HDL Operations/Bit Concat  numInputs=2
  Bit Slice : hdlsllib/HDL Operations/Bit Slice  lidx=15  ridx=0
  Bit Slice1 : hdlsllib/HDL Operations/Bit Slice  lidx=31  ridx=16
  Data Type Conversion : DataTypeConversion  OutDataTypeStr=int16  ConvertRealWorld=Stored Integer (SI)
  Data Type Conversion1 : DataTypeConversion  OutDataTypeStr=int16  ConvertRealWorld=Stored Integer (SI)
  Gain : Gain  Gain=1/10  OutDataTypeStr=int16
  Gain1 : Gain  Gain=1/10  OutDataTypeStr=int16
  iq_scale_scope : Scope  NumInputPorts=2
  Out1 : Outport
  wires:
  Gain1/1 -> Bit Concat/2, iq_scale_scope/1
  In1/1 -> Bit Slice1/1, Bit Slice/1
  Bit Slice/1 -> Data Type Conversion/1
  Data Type Conversion/1 -> Gain/1
  Data Type Conversion1/1 -> Gain1/1
  Bit Concat/1 -> Out1/1
  Gain/1 -> Bit Concat/1, iq_scale_scope/2
  Bit Slice1/1 -> Data Type Conversion1/1

== system CryoDetHcd/DspCore/DSP/scale2 ==
  In1 : Inport
  Bit Concat : hdlsllib/HDL Operations/Bit Concat  numInputs=2
  Bit Slice : hdlsllib/HDL Operations/Bit Slice  lidx=15  ridx=0
  Bit Slice1 : hdlsllib/HDL Operations/Bit Slice  lidx=31  ridx=16
  Data Type Conversion : DataTypeConversion  OutDataTypeStr=int16  ConvertRealWorld=Stored Integer (SI)
  Data Type Conversion1 : DataTypeConversion  OutDataTypeStr=int16  ConvertRealWorld=Stored Integer (SI)
  Gain : Gain  Gain=1/10  OutDataTypeStr=int16
  Gain1 : Gain  Gain=1/10  OutDataTypeStr=int16
  iq_scale_scope : Scope  NumInputPorts=2
  Out1 : Outport
  wires:
  Bit Slice1/1 -> Data Type Conversion1/1
  Gain/1 -> iq_scale_scope/2, Bit Concat/1
  Bit Concat/1 -> Out1/1
  Data Type Conversion1/1 -> Gain1/1
  Data Type Conversion/1 -> Gain/1
  Bit Slice/1 -> Data Type Conversion/1
  In1/1 -> Bit Slice/1, Bit Slice1/1
  Gain1/1 -> iq_scale_scope/1, Bit Concat/2

== system CryoDetHcd/DspCore/DSP/Synthesis_pipelined/Synthesis ==
  valid : Inport
  im0 : Inport  Port=2
  re0 : Inport  Port=3
  im1 : Inport  Port=4
  re1 : Inport  Port=5
  im2 : Inport  Port=6
  re2 : Inport  Port=7
  im3 : Inport  Port=8
  re3 : Inport  Port=9
  scale_select : Inport  Port=10
  Combine : Subsystem
  Post_synthesis0 : Subsystem
  Post_sytnehsis1 : Subsystem
  Syntehsis0 : Subsystem
  Syntehsis1 : Subsystem
  im : Outport
  re : Outport  Port=2
  wires:
  Syntehsis0/1(valid_o) -> Post_synthesis0/1(valid)
  Combine/3(re_o) -> re/1
  Post_sytnehsis1/3(reo) -> Combine/5(re1)
  Post_sytnehsis1/2(im0) -> Combine/4(im1)
  Post_synthesis0/3(reo) -> Combine/3(re0)
  Post_synthesis0/2(im0) -> Combine/2(im0)
  Post_synthesis0/1(valid0) -> Combine/1(valid)
  Syntehsis0/3(re0) -> Post_synthesis0/3(re)
  Syntehsis0/2(im0) -> Post_synthesis0/2(im)
  Syntehsis1/1(valid_o) -> Post_sytnehsis1/1(valid)
  Syntehsis1/3(re0) -> Post_sytnehsis1/3(re)
  Syntehsis1/2(im0) -> Post_sytnehsis1/2(im)
  im3/1 -> Syntehsis1/4(imag_i1)
  re1/1 -> Syntehsis0/5(real_i1)
  valid/1 -> Syntehsis1/3(valid_i), Syntehsis0/3(valid_i)
  re3/1 -> Syntehsis1/5(real_i1)
  im1/1 -> Syntehsis0/4(imag_i1)
  im0/1 -> Syntehsis0/1(imag_i0)
  re0/1 -> Syntehsis0/2(real_i0)
  re2/1 -> Syntehsis1/2(real_i0)
  im2/1 -> Syntehsis1/1(imag_i0)
  Combine/2(im_o) -> im/1
  scale_select/1 -> Syntehsis1/6(scale_seelct), Syntehsis0/6(scale_seelct)
